simulink model "Grid_SensorLayout_SpatialAllignment_Clustering"  (R2018a)
settings: Solver=FixedStepAuto  StartTime=0.0  StopTime=SimulationTime  FixedStep=SamplingTime  RelTol=1e-3
values from neighbouring files (symbols this model uses):
  ValidateGRID = true    [SensorFusion_Script0_main.m]
  ValidateLAYOUT = true    [SensorFusion_Script0_main.m]
  VisualizeCLUSTERING = true    [SensorFusion_Script0_main.m]
undefined symbols (not defined in the file or in its folder): ACTIVATE_CAM, ACTIVATE_RAD, CAM1_detTimeStamp, CAM1_MeasNoise, CAM1_objClassID, CAM1_PX, CAM1_PY, CAM1_VX, CAM1_VY, CAM2_detTimeStamp, CAM2_MeasNoise, CAM2_objClassID, CAM2_PX, CAM2_PY, CAM2_VX, CAM2_VY, CAM3_detTimeStamp, CAM3_MeasNoise, CAM3_objClassID, CAM3_PX, CAM3_PY, CAM3_VX, CAM3_VY, CAM4_detTimeStamp, CAM4_MeasNoise, CAM4_objClassID, CAM4_PX, CAM4_PY, CAM4_VX, CAM4_VY, CAM5_detTimeStamp, CAM5_MeasNoise, CAM5_objClassID, CAM5_PX, CAM5_PY, CAM5_VX, CAM5_VY, CAM6_detTimeStamp, CAM6_MeasNoise, CAM6_objClassID, CAM6_PX, CAM6_PY, CAM6_VX, CAM6_VY, CAM7_detTimeStamp, CAM7_MeasNoise, CAM7_objClassID, CAM7_PX, CAM7_PY, CAM7_VX, CAM7_VY, CAM8_detTimeStamp, CAM8_MeasNoise, CAM8_objClassID, CAM8_PX, CAM8_PY, CAM8_VX, CAM8_VY, CAM_nMeas, CAM_TYPE ... (+171)
libraries: simulink_extras x4
(part 6 of 10)

== system Grid_SensorLayout_SpatialAllignment_Clustering/SENSOR_MEASUREMENTS/RADAR_CAMERA_EGO_SENSOR_INTERFACE/RadarSensors/Radar4/Subsystem ==
  SensorData : Inport
  px : Inport  Port=2
  py : Inport  Port=3
  vx : Inport  Port=4
  vy : Inport  Port=5
  id : Inport  Port=6
  SNR : Inport  Port=7
  NOISE_COV : Inport  Port=8
  TIME_STAMP : Inport  Port=9
  iter : Inport  Port=10
  Assignment : Assignment  DiagnosticForDimensions=Warning  IndexOptions=Index vector (port)  Indices=1  OutputSizes=1
  Bus Creator1 : BusCreator  Inputs=12  OutDataTypeStr=Bus: RadarMeasParam  NonVirtualBus=on
  Bus Creator2 : BusCreator  Inputs=12  OutDataTypeStr=Bus: RadarMeasParam  NonVirtualBus=on
  Constant{,1..5,8} (7 alike) : Constant  Value=single(0)
  Constant10 : Constant  Value=single(zeros(4,4))
  Constant13 : Constant  Value=single(10)
  Constant14 : Constant  Value=uint8(4)
  Constant16 : Constant  Value=int16(-1)
  Constant17 : Constant  Value=boolean(0)  OutDataTypeStr=boolean
  Constant6 : Constant  Value=uint8(4)
  Constant7 : Constant  Value=int16(0)
  Constant9 : Constant  Value=boolean(0)  OutDataTypeStr=boolean
  Switch : Switch  Criteria=u2 ~= 0
  R4 : Outport
  wires:
  Switch/1 -> Assignment/2
  Bus Creator2/1 -> Switch/1
  Bus Creator1/1 -> Switch/3
  Assignment/1 -> R4/1
  Constant5/1 -> Bus Creator1/9  "SNR"
  iter/1 -> Assignment/3
  id/1 -> Bus Creator1/2, Bus Creator2/2, Switch/2  "measID"
  SensorData/1 -> Assignment/1
  Constant3/1 -> Bus Creator1/7  "vy"
  Constant2/1 -> Bus Creator1/6  "vx"
  Constant1/1 -> Bus Creator1/5  "py"
  Constant/1 -> Bus Creator1/4  "px"
  Constant6/1 -> Bus Creator1/3  "radarID"
  TIME_STAMP/1 -> Bus Creator2/1  "TimeStamp"
  Constant14/1 -> Bus Creator2/3  "radarID"
  px/1 -> Bus Creator2/4  "px"
  py/1 -> Bus Creator2/5  "py"
  vx/1 -> Bus Creator2/6  "vx"
  vy/1 -> Bus Creator2/7  "vy"
  NOISE_COV/1 -> Bus Creator2/8  "NoiseCovarience"
  SNR/1 -> Bus Creator2/9  "SNR"
  Constant17/1 -> Bus Creator2/12  "StationaryFlag"
  Constant13/1 -> Bus Creator2/11  "measConfidence"
  Constant16/1 -> Bus Creator2/10  "Classification"
  Constant9/1 -> Bus Creator1/12  "StationaryFlag"
  Constant4/1 -> Bus Creator1/11  "measConfidence"
  Constant7/1 -> Bus Creator1/10  "Classification"
  Constant8/1 -> Bus Creator1/1  "TimeStamp"
  Constant10/1 -> Bus Creator1/8  "NoiseCovarience"

== system Grid_SensorLayout_SpatialAllignment_Clustering/SENSOR_MEASUREMENTS/RADAR_CAMERA_EGO_SENSOR_INTERFACE/RadarSensors/Radar5/ExtractMeasParam ==
  idx : Inport
  time : Inport  Port=2
  Constant : Constant  Value=RAD5_PX
  Constant1 : Constant  Value=RAD5_PY
  Constant2 : Constant  Value=RAD5_VX
  Constant3 : Constant  Value=RAD5_VY
  Constant4 : Constant  Value=RAD5_SNR
  Constant5 : Constant  Value=RAD5_MeasNoise
  Constant6 : Constant  Value=RAD5_detTimeStamp
  MeasNoise : Selector  NumberOfDimensions=4  InputPortWidth=3  IndexOptions=Index vector (port),Select all,Select all,Index vector (port)  Indices=[1 3],1,1,1  OutputSizes=1,1,1,1
  PosX : Selector  NumberOfDimensions=2  InputPortWidth=3  IndexOptions=Index vector (port),Index vector (port)  Indices=[1 3],1  OutputSizes=1,1
  PosY : Selector  NumberOfDimensions=2  InputPortWidth=3  IndexOptions=Index vector (port),Index vector (port)  Indices=[1 3],1  OutputSizes=1,1
  Reshape : Reshape  OutputDimensionality=Customize  OutputDimensions=[4,4]
  VelX : Selector  NumberOfDimensions=2  InputPortWidth=3  IndexOptions=Index vector (port),Index vector (port)  Indices=[1 3],1  OutputSizes=1,1
  VelY : Selector  NumberOfDimensions=2  InputPortWidth=3  IndexOptions=Index vector (port),Index vector (port)  Indices=[1 3],1  OutputSizes=1,1
  snr : Selector  NumberOfDimensions=2  InputPortWidth=3  IndexOptions=Index vector (port),Index vector (port)  Indices=[1 3],1  OutputSizes=1,1
  timeStamp : Selector  NumberOfDimensions=2  InputPortWidth=3  IndexOptions=Select all,Index vector (port)  Indices=[1 3],1  OutputSizes=1,1
  PX : Outport
  PY : Outport  Port=2
  VX : Outport  Port=3
  VY : Outport  Port=4
  SNR : Outport  Port=5
  NOISE_COV : Outport  Port=6
  measCaptureTime : Outport  Port=7
  wires:
  Constant3/1 -> VelY/1
  Constant2/1 -> VelX/1
  VelY/1 -> VY/1
  Constant/1 -> PosX/1
  idx/1 -> MeasNoise/3, snr/3, VelY/3, VelX/3, PosY/3, PosX/3
  Constant1/1 -> PosY/1
  VelX/1 -> VX/1
  PosX/1 -> PX/1
  PosY/1 -> PY/1
  time/1 -> timeStamp/2, MeasNoise/2, snr/2, VelY/2, VelX/2, PosY/2, PosX/2
  Constant4/1 -> snr/1
  snr/1 -> SNR/1
  Constant5/1 -> MeasNoise/1
  Constant6/1 -> timeStamp/1
  MeasNoise/1 -> Reshape/1
  timeStamp/1 -> measCaptureTime/1
  Reshape/1 -> NOISE_COV/1

== system Grid_SensorLayout_SpatialAllignment_Clustering/SENSOR_MEASUREMENTS/RADAR_CAMERA_EGO_SENSOR_INTERFACE/RadarSensors/Radar5/IsValid1 ==
  idx : Inport
  px : Inport  Port=2
  py : Inport  Port=3
  vx : Inport  Port=4
  vy : Inport  Port=5
  Abs{,1..3} (4 alike) : Abs
  Add : Sum  Inputs=++++
  Constant : Constant  Value=uint16(0)
  Data Type Conversion : DataTypeConversion  OutDataTypeStr=uint16
  Switch : Switch  Threshold=0.0001
  ID : Outport
  wires:
  Add/1 -> Switch/2
  Abs2/1 -> Add/3
  Constant/1 -> Switch/3
  Abs/1 -> Add/1
  px/1 -> Abs/1
  Abs3/1 -> Add/4
  Abs1/1 -> Add/2
  vy/1 -> Abs3/1
  py/1 -> Abs1/1
  vx/1 -> Abs2/1
  idx/1 -> Data Type Conversion/1
  Switch/1 -> ID/1
  Data Type Conversion/1 -> Switch/1

== system Grid_SensorLayout_SpatialAllignment_Clustering/SENSOR_MEASUREMENTS/RADAR_CAMERA_EGO_SENSOR_INTERFACE/RadarSensors/Radar5/Subsystem ==
  SensorData : Inport
  px : Inport  Port=2
  py : Inport  Port=3
  vx : Inport  Port=4
  vy : Inport  Port=5
  id : Inport  Port=6
  SNR : Inport  Port=7
  NOISE_COV : Inport  Port=8
  TIME_STAMP : Inport  Port=9
  iter : Inport  Port=10
  Assignment : Assignment  DiagnosticForDimensions=Warning  IndexOptions=Index vector (port)  Indices=1  OutputSizes=1
  Bus Creator1 : BusCreator  Inputs=12  OutDataTypeStr=Bus: RadarMeasParam  NonVirtualBus=on
  Bus Creator2 : BusCreator  Inputs=12  OutDataTypeStr=Bus: RadarMeasParam  NonVirtualBus=on
  Constant{,1..5,8} (7 alike) : Constant  Value=single(0)
  Constant10 : Constant  Value=single(zeros(4,4))
  Constant13 : Constant  Value=single(10)
  Constant14 : Constant  Value=uint8(5)
  Constant16 : Constant  Value=int16(-1)
  Constant17 : Constant  Value=boolean(0)  OutDataTypeStr=boolean
  Constant6 : Constant  Value=uint8(5)
  Constant7 : Constant  Value=int16(0)
  Constant9 : Constant  Value=boolean(0)  OutDataTypeStr=boolean
  Switch : Switch  Criteria=u2 ~= 0
  R5 : Outport
  wires:
  Switch/1 -> Assignment/2
  Bus Creator2/1 -> Switch/1
  Bus Creator1/1 -> Switch/3
  Assignment/1 -> R5/1
  Constant5/1 -> Bus Creator1/9  "SNR"
  iter/1 -> Assignment/3
  id/1 -> Bus Creator1/2, Bus Creator2/2, Switch/2  "measID"
  SensorData/1 -> Assignment/1
  Constant3/1 -> Bus Creator1/7  "vy"
  Constant2/1 -> Bus Creator1/6  "vx"
  Constant1/1 -> Bus Creator1/5  "py"
  Constant/1 -> Bus Creator1/4  "px"
  Constant6/1 -> Bus Creator1/3  "radarID"
  TIME_STAMP/1 -> Bus Creator2/1  "TimeStamp"
  Constant14/1 -> Bus Creator2/3  "radarID"
  px/1 -> Bus Creator2/4  "px"
  py/1 -> Bus Creator2/5  "py"
  vx/1 -> Bus Creator2/6  "vx"
  vy/1 -> Bus Creator2/7  "vy"
  NOISE_COV/1 -> Bus Creator2/8  "NoiseCovarience"
  SNR/1 -> Bus Creator2/9  "SNR"
  Constant17/1 -> Bus Creator2/12  "StationaryFlag"
  Constant13/1 -> Bus Creator2/11  "measConfidence"
  Constant16/1 -> Bus Creator2/10  "Classification"
  Constant9/1 -> Bus Creator1/12  "StationaryFlag"
  Constant4/1 -> Bus Creator1/11  "measConfidence"
  Constant7/1 -> Bus Creator1/10  "Classification"
  Constant8/1 -> Bus Creator1/1  "TimeStamp"
  Constant10/1 -> Bus Creator1/8  "NoiseCovarience"

== system Grid_SensorLayout_SpatialAllignment_Clustering/SENSOR_MEASUREMENTS/RADAR_CAMERA_EGO_SENSOR_INTERFACE/RadarSensors/Radar6/ExtractMeasParam ==
  idx : Inport
  time : Inport  Port=2
  Constant : Constant  Value=RAD6_PX
  Constant1 : Constant  Value=RAD6_PY
  Constant2 : Constant  Value=RAD6_VX
  Constant3 : Constant  Value=RAD6_VY
  Constant4 : Constant  Value=RAD6_SNR
  Constant5 : Constant  Value=RAD6_MeasNoise
  Constant6 : Constant  Value=RAD6_detTimeStamp
  MeasNoise : Selector  NumberOfDimensions=4  InputPortWidth=3  IndexOptions=Index vector (port),Select all,Select all,Index vector (port)  Indices=[1 3],1,1,1  OutputSizes=1,1,1,1
  PosX : Selector  NumberOfDimensions=2  InputPortWidth=3  IndexOptions=Index vector (port),Index vector (port)  Indices=[1 3],1  OutputSizes=1,1
  PosY : Selector  NumberOfDimensions=2  InputPortWidth=3  IndexOptions=Index vector (port),Index vector (port)  Indices=[1 3],1  OutputSizes=1,1
  Reshape : Reshape  OutputDimensionality=Customize  OutputDimensions=[4,4]
  VelX : Selector  NumberOfDimensions=2  InputPortWidth=3  IndexOptions=Index vector (port),Index vector (port)  Indices=[1 3],1  OutputSizes=1,1
  VelY : Selector  NumberOfDimensions=2  InputPortWidth=3  IndexOptions=Index vector (port),Index vector (port)  Indices=[1 3],1  OutputSizes=1,1
  snr : Selector  NumberOfDimensions=2  InputPortWidth=3  IndexOptions=Index vector (port),Index vector (port)  Indices=[1 3],1  OutputSizes=1,1
  timeStamp : Selector  NumberOfDimensions=2  InputPortWidth=3  IndexOptions=Select all,Index vector (port)  Indices=[1 3],1  OutputSizes=1,1
  PX : Outport
  PY : Outport  Port=2
  VX : Outport  Port=3
  VY : Outport  Port=4
  SNR : Outport  Port=5
  NOISE_COV : Outport  Port=6
  measCaptureTime : Outport  Port=7
  wires:
  Constant3/1 -> VelY/1
  Constant2/1 -> VelX/1
  VelY/1 -> VY/1
  Constant/1 -> PosX/1
  idx/1 -> MeasNoise/3, snr/3, VelY/3, VelX/3, PosY/3, PosX/3
  Constant1/1 -> PosY/1
  VelX/1 -> VX/1
  PosX/1 -> PX/1
  PosY/1 -> PY/1
  time/1 -> timeStamp/2, MeasNoise/2, snr/2, VelY/2, VelX/2, PosY/2, PosX/2
  Constant4/1 -> snr/1
  snr/1 -> SNR/1
  Constant5/1 -> MeasNoise/1
  Constant6/1 -> timeStamp/1
  MeasNoise/1 -> Reshape/1
  timeStamp/1 -> measCaptureTime/1
  Reshape/1 -> NOISE_COV/1

== system Grid_SensorLayout_SpatialAllignment_Clustering/SENSOR_MEASUREMENTS/RADAR_CAMERA_EGO_SENSOR_INTERFACE/RadarSensors/Radar6/IsValid1 ==
  idx : Inport
  px : Inport  Port=2
  py : Inport  Port=3
  vx : Inport  Port=4
  vy : Inport  Port=5
  Abs{,1..3} (4 alike) : Abs
  Add : Sum  Inputs=++++
  Constant : Constant  Value=uint16(0)
  Data Type Conversion : DataTypeConversion  OutDataTypeStr=uint16
  Switch : Switch  Threshold=0.0001
  ID : Outport
  wires:
  Add/1 -> Switch/2
  Abs2/1 -> Add/3
  Constant/1 -> Switch/3
  Abs/1 -> Add/1
  px/1 -> Abs/1
  Abs3/1 -> Add/4
  Abs1/1 -> Add/2
  vy/1 -> Abs3/1
  py/1 -> Abs1/1
  vx/1 -> Abs2/1
  idx/1 -> Data Type Conversion/1
  Switch/1 -> ID/1
  Data Type Conversion/1 -> Switch/1

== system Grid_SensorLayout_SpatialAllignment_Clustering/SENSOR_MEASUREMENTS/RADAR_CAMERA_EGO_SENSOR_INTERFACE/RadarSensors/Radar6/Subsystem ==
  SensorData : Inport
  px : Inport  Port=2
  py : Inport  Port=3
  vx : Inport  Port=4
  vy : Inport  Port=5
  id : Inport  Port=6
  SNR : Inport  Port=7
  NOISE_COV : Inport  Port=8
  TIME_STAMP : Inport  Port=9
  iter : Inport  Port=10
  Assignment : Assignment  DiagnosticForDimensions=Warning  IndexOptions=Index vector (port)  Indices=1  OutputSizes=1
  Bus Creator1 : BusCreator  Inputs=12  OutDataTypeStr=Bus: RadarMeasParam  NonVirtualBus=on
  Bus Creator2 : BusCreator  Inputs=12  OutDataTypeStr=Bus: RadarMeasParam  NonVirtualBus=on
  Constant{,1..5,8} (7 alike) : Constant  Value=single(0)
  Constant10 : Constant  Value=single(zeros(4,4))
  Constant13 : Constant  Value=single(10)
  Constant14 : Constant  Value=uint8(6)
  Constant16 : Constant  Value=int16(-1)
  Constant17 : Constant  Value=boolean(0)  OutDataTypeStr=boolean
  Constant6 : Constant  Value=uint8(6)
  Constant7 : Constant  Value=int16(0)
  Constant9 : Constant  Value=boolean(0)  OutDataTypeStr=boolean
  Switch : Switch  Criteria=u2 ~= 0
  R6 : Outport
  wires:
  Switch/1 -> Assignment/2
  Bus Creator2/1 -> Switch/1
  Bus Creator1/1 -> Switch/3
  Assignment/1 -> R6/1
  Constant5/1 -> Bus Creator1/9  "SNR"
  iter/1 -> Assignment/3
  id/1 -> Bus Creator1/2, Bus Creator2/2, Switch/2  "measID"
  SensorData/1 -> Assignment/1
  Constant3/1 -> Bus Creator1/7  "vy"
  Constant2/1 -> Bus Creator1/6  "vx"
  Constant1/1 -> Bus Creator1/5  "py"
  Constant/1 -> Bus Creator1/4  "px"
  Constant6/1 -> Bus Creator1/3  "radarID"
  TIME_STAMP/1 -> Bus Creator2/1  "TimeStamp"
  Constant14/1 -> Bus Creator2/3  "radarID"
  px/1 -> Bus Creator2/4  "px"
  py/1 -> Bus Creator2/5  "py"
  vx/1 -> Bus Creator2/6  "vx"
  vy/1 -> Bus Creator2/7  "vy"
  NOISE_COV/1 -> Bus Creator2/8  "NoiseCovarience"
  SNR/1 -> Bus Creator2/9  "SNR"
  Constant17/1 -> Bus Creator2/12  "StationaryFlag"
  Constant13/1 -> Bus Creator2/11  "measConfidence"
  Constant16/1 -> Bus Creator2/10  "Classification"
  Constant9/1 -> Bus Creator1/12  "StationaryFlag"
  Constant4/1 -> Bus Creator1/11  "measConfidence"
  Constant7/1 -> Bus Creator1/10  "Classification"
  Constant8/1 -> Bus Creator1/1  "TimeStamp"
  Constant10/1 -> Bus Creator1/8  "NoiseCovarience"

== system Grid_SensorLayout_SpatialAllignment_Clustering/SENSOR_MEASUREMENTS/RADAR_CAMERA_EGO_SENSOR_INTERFACE/RoadSensors/LineSensor1/CHECK_IF_DATA_IS_VALID ==
  LineID : Inport
  curvature : Inport  Port=2
  curvatureRate : Inport  Port=3
  curvLength : Inport  Port=4
  HeadingAngle : Inport  Port=5
  Abs{,1..3} (4 alike) : Abs
  Add : Sum  Inputs=++++
  Constant : Constant  Value=uint16(0)
  Data Type Conversion : DataTypeConversion  OutDataTypeStr=uint16
  Switch : Switch  Threshold=0.000001
  validID : Outport
  wires:
  Add/1 -> Switch/2
  Abs2/1 -> Add/3
  Constant/1 -> Switch/3
  Abs/1 -> Add/1
  curvature/1 -> Abs/1
  Abs3/1 -> Add/4
  Abs1/1 -> Add/2
  HeadingAngle/1 -> Abs3/1
  curvatureRate/1 -> Abs1/1
  curvLength/1 -> Abs2/1
  LineID/1 -> Data Type Conversion/1
  Switch/1 -> validID/1
  Data Type Conversion/1 -> Switch/1

== system Grid_SensorLayout_SpatialAllignment_Clustering/SENSOR_MEASUREMENTS/RADAR_CAMERA_EGO_SENSOR_INTERFACE/RoadSensors/LineSensor1/GET_DATA ==
  idx : Inport
  time : Inport  Port=2
  Constant : Constant  Value=LINE_CURVATURE_CAM1
  Constant1 : Constant  Value=LINE_CURVDERIVATIVE_CAM1
  Constant2 : Constant  Value=LINE_CURVELENGTH_CAM1
  Constant3 : Constant  Value=LINE_HEADINGANGLE_CAM1
  Constant4 : Constant  Value=LINE_LATERALOFFSET_CAM1
  Constant5 : Constant  Value=LINE_XMIN_CAM1
  Constant6 : Constant  Value=LINE_detTimeStamp_CAM1
  Constant7 : Constant  Value=LINE_XMAX_CAM1
  Constant8 : Constant  Value=LINE_WIDTH_CAM1
  CurvLength : Selector  NumberOfDimensions=2  InputPortWidth=3  IndexOptions=Index vector (port),Index vector (port)  Indices=[1 3],1  OutputSizes=1,1
  Curvature : Selector  NumberOfDimensions=2  InputPortWidth=3  IndexOptions=Index vector (port),Index vector (port)  Indices=[1 3],1  OutputSizes=1,1
  CurvatureRate : Selector  NumberOfDimensions=2  InputPortWidth=3  IndexOptions=Index vector (port),Index vector (port)  Indices=[1 3],1  OutputSizes=1,1
  HeadingAngle : Selector  NumberOfDimensions=2  InputPortWidth=3  IndexOptions=Index vector (port),Index vector (port)  Indices=[1 3],1  OutputSizes=1,1
  LateralOffset : Selector  NumberOfDimensions=2  InputPortWidth=3  IndexOptions=Index vector (port),Index vector (port)  Indices=[1 3],1  OutputSizes=1,1
  lineWidth : Selector  NumberOfDimensions=2  InputPortWidth=3  IndexOptions=Index vector (port),Index vector (port)  Indices=[1 3],1  OutputSizes=1,1
  minValidX : Selector  NumberOfDimensions=2  InputPortWidth=3  IndexOptions=Index vector (port),Index vector (port)  Indices=[1 3],1  OutputSizes=1,1
  minValidY : Selector  NumberOfDimensions=2  InputPortWidth=3  IndexOptions=Index vector (port),Index vector (port)  Indices=[1 3],1  OutputSizes=1,1
  timeStamp : Selector  NumberOfDimensions=2  InputPortWidth=3  IndexOptions=Select all,Index vector (port)  Indices=[1 3],1  OutputSizes=1,1
  curvature : Outport
  curvRate : Outport  Port=2
  curvLength : Outport  Port=3
  headingAngle : Outport  Port=4
  lateralOffset : Outport  Port=5
  xmin : Outport  Port=6
  xmax : Outport  Port=7
  lineMarkWidth : Outport  Port=8
  measCaptureTime : Outport  Port=9
  wires:
  Constant3/1 -> HeadingAngle/1
  Constant2/1 -> CurvLength/1
  HeadingAngle/1 -> headingAngle/1
  Constant/1 -> Curvature/1
  Constant1/1 -> CurvatureRate/1
  CurvLength/1 -> curvLength/1
  Curvature/1 -> curvature/1
  CurvatureRate/1 -> curvRate/1
  Constant4/1 -> LateralOffset/1
  Constant5/1 -> minValidX/1
  Constant6/1 -> timeStamp/1
  timeStamp/1 -> measCaptureTime/1
  minValidX/1 -> xmin/1
  LateralOffset/1 -> lateralOffset/1
  minValidY/1 -> xmax/1
  Constant7/1 -> minValidY/1
  lineWidth/1 -> lineMarkWidth/1
  time/1 -> minValidX/2, minValidY/2, lineWidth/2, timeStamp/2, LateralOffset/2, HeadingAngle/2, CurvLength/2, CurvatureRate/2, Curvature/2
  idx/1 -> minValidX/3, lineWidth/3, minValidY/3, LateralOffset/3, HeadingAngle/3, CurvLength/3, CurvatureRate/3, Curvature/3
  Constant8/1 -> lineWidth/1

== system Grid_SensorLayout_SpatialAllignment_Clustering/SENSOR_MEASUREMENTS/RADAR_CAMERA_EGO_SENSOR_INTERFACE/RoadSensors/LineSensor1/SET_DATA ==
  CameraLineCoeff : Inport
  curv : Inport  Port=2
  curvRate : Inport  Port=3
  curvLen : Inport  Port=4
  alpha : Inport  Port=5
  ValidID : Inport  Port=6
  lateralOffset : Inport  Port=7
  xmin : Inport  Port=8
  xmax : Inport  Port=9
  lineWidth : Inport  Port=10
  TIME_STAMP : Inport  Port=11
  iter : Inport  Port=12
  Assignment : Assignment  DiagnosticForDimensions=Warning  IndexOptions=Index vector (port)  Indices=1  OutputSizes=1
  Bus Creator1 : BusCreator  Inputs=11  OutDataTypeStr=Bus: LineMeasParam  NonVirtualBus=on
  Bus Creator2 : BusCreator  Inputs=11  OutDataTypeStr=Bus: LineMeasParam  NonVirtualBus=on
  Constant1 : Constant  Value=single(10)
  Constant14 : Constant  Value=uint8(1)
  Constant2 : Constant  Value=single(10)
  Constant{35..39,43} (6 alike) : Constant  Value=single(0)
  Constant44 : Constant  Value=single(10)
  Switch : Switch  Criteria=u2 ~= 0
  C1 : Outport
  wires:
  Bus Creator1/1 -> Switch/3
  ValidID/1 -> Bus Creator1/2, Switch/2, Bus Creator2/2  "lineID"
  Bus Creator2/1 -> Switch/1
  CameraLineCoeff/1 -> Assignment/1
  Switch/1 -> Assignment/2
  iter/1 -> Assignment/3
  Assignment/1 -> C1/1
  TIME_STAMP/1 -> Bus Creator2/1  "TimeStamp"
  curv/1 -> Bus Creator2/4  "curvature"
  curvRate/1 -> Bus Creator2/5  "curvatureRate"
  curvLen/1 -> Bus Creator2/6  "curveLength"
  alpha/1 -> Bus Creator2/7  "HeadingAngle"
  lateralOffset/1 -> Bus Creator2/8  "LateralOffset"
  lineWidth/1 -> Bus Creator2/11  "LineMarkWidth"
  xmax/1 -> Bus Creator2/10  "validMinLongCoordLine"
  xmin/1 -> Bus Creator2/9  "validMaxLongCoordLine"
  Constant35/1 -> Bus Creator1/1  "TimeStamp"
  Constant14/1 -> Bus Creator2/3, Bus Creator1/3  "cameraID"
  Constant36/1 -> Bus Creator1/4  "curvature"
  Constant37/1 -> Bus Creator1/5  "curvatureRate"
  Constant38/1 -> Bus Creator1/6  "curveLength"
  Constant39/1 -> Bus Creator1/7  "HeadingAngle"
  Constant43/1 -> Bus Creator1/8  "LateralOffset"
  Constant44/1 -> Bus Creator1/9  "validMaxLongCoordLine"
  Constant1/1 -> Bus Creator1/10  "validMinLongCoordLine"
  Constant2/1 -> Bus Creator1/11  "LineMarkWidth"

== system Grid_SensorLayout_SpatialAllignment_Clustering/SENSOR_MEASUREMENTS/RADAR_CAMERA_EGO_SENSOR_INTERFACE/RoadSensors/LineSensor2/ExtractMeasParam1 ==
  idx : Inport
  time : Inport  Port=2
  Constant : Constant  Value=LINE_CURVATURE_CAM2
  Constant1 : Constant  Value=LINE_CURVDERIVATIVE_CAM2
  Constant2 : Constant  Value=LINE_CURVELENGTH_CAM2
  Constant3 : Constant  Value=LINE_HEADINGANGLE_CAM2
  Constant4 : Constant  Value=LINE_LATERALOFFSET_CAM2
  Constant5 : Constant  Value=LINE_XMIN_CAM2
  Constant6 : Constant  Value=LINE_detTimeStamp_CAM2
  Constant7 : Constant  Value=LINE_XMAX_CAM2
  Constant8 : Constant  Value=LINE_WIDTH_CAM2
  CurvLength : Selector  NumberOfDimensions=2  InputPortWidth=3  IndexOptions=Index vector (port),Index vector (port)  Indices=[1 3],1  OutputSizes=1,1
  Curvature : Selector  NumberOfDimensions=2  InputPortWidth=3  IndexOptions=Index vector (port),Index vector (port)  Indices=[1 3],1  OutputSizes=1,1
  CurvatureRate : Selector  NumberOfDimensions=2  InputPortWidth=3  IndexOptions=Index vector (port),Index vector (port)  Indices=[1 3],1  OutputSizes=1,1
  HeadingAngle : Selector  NumberOfDimensions=2  InputPortWidth=3  IndexOptions=Index vector (port),Index vector (port)  Indices=[1 3],1  OutputSizes=1,1
  LateralOffset : Selector  NumberOfDimensions=2  InputPortWidth=3  IndexOptions=Index vector (port),Index vector (port)  Indices=[1 3],1  OutputSizes=1,1
  lineWidth : Selector  NumberOfDimensions=2  InputPortWidth=3  IndexOptions=Index vector (port),Index vector (port)  Indices=[1 3],1  OutputSizes=1,1
  minValidX : Selector  NumberOfDimensions=2  InputPortWidth=3  IndexOptions=Index vector (port),Index vector (port)  Indices=[1 3],1  OutputSizes=1,1
  minValidY : Selector  NumberOfDimensions=2  InputPortWidth=3  IndexOptions=Index vector (port),Index vector (port)  Indices=[1 3],1  OutputSizes=1,1
  timeStamp : Selector  NumberOfDimensions=2  InputPortWidth=3  IndexOptions=Select all,Index vector (port)  Indices=[1 3],1  OutputSizes=1,1
  curvature : Outport
  curvRate : Outport  Port=2
  curvLength : Outport  Port=3
  headingAngle : Outport  Port=4
  lateralOffset : Outport  Port=5
  xmin : Outport  Port=6
  xmax : Outport  Port=7
  lineMarkWidth : Outport  Port=8
  measCaptureTime : Outport  Port=9
  wires:
  Constant3/1 -> HeadingAngle/1
  Constant2/1 -> CurvLength/1
  HeadingAngle/1 -> headingAngle/1
  Constant/1 -> Curvature/1
  Constant1/1 -> CurvatureRate/1
  CurvLength/1 -> curvLength/1
  Curvature/1 -> curvature/1
  CurvatureRate/1 -> curvRate/1
  Constant4/1 -> LateralOffset/1
  Constant5/1 -> minValidX/1
  Constant6/1 -> timeStamp/1
  timeStamp/1 -> measCaptureTime/1
  minValidX/1 -> xmin/1
  LateralOffset/1 -> lateralOffset/1
  minValidY/1 -> xmax/1
  Constant7/1 -> minValidY/1
  lineWidth/1 -> lineMarkWidth/1
  time/1 -> minValidX/2, minValidY/2, lineWidth/2, timeStamp/2, LateralOffset/2, HeadingAngle/2, CurvLength/2, CurvatureRate/2, Curvature/2
  idx/1 -> minValidX/3, lineWidth/3, minValidY/3, LateralOffset/3, HeadingAngle/3, CurvLength/3, CurvatureRate/3, Curvature/3
  Constant8/1 -> lineWidth/1

== system Grid_SensorLayout_SpatialAllignment_Clustering/SENSOR_MEASUREMENTS/RADAR_CAMERA_EGO_SENSOR_INTERFACE/RoadSensors/LineSensor2/IsValid2 ==
  LineID : Inport
  curvature : Inport  Port=2
  curvatureRate : Inport  Port=3
  curvLength : Inport  Port=4
  HeadingAngle : Inport  Port=5
  Abs{,1..3} (4 alike) : Abs
  Add : Sum  Inputs=++++
  Constant : Constant  Value=uint16(0)
  Data Type Conversion : DataTypeConversion  OutDataTypeStr=uint16
  Switch : Switch  Threshold=0.000001
  validID : Outport
  wires:
  Add/1 -> Switch/2
  Abs2/1 -> Add/3
  Constant/1 -> Switch/3
  Abs/1 -> Add/1
  curvature/1 -> Abs/1
  Abs3/1 -> Add/4
  Abs1/1 -> Add/2
  HeadingAngle/1 -> Abs3/1
  curvatureRate/1 -> Abs1/1
  curvLength/1 -> Abs2/1
  LineID/1 -> Data Type Conversion/1
  Switch/1 -> validID/1
  Data Type Conversion/1 -> Switch/1

== system Grid_SensorLayout_SpatialAllignment_Clustering/SENSOR_MEASUREMENTS/RADAR_CAMERA_EGO_SENSOR_INTERFACE/RoadSensors/LineSensor2/Subsystem1 ==
  CameraLineCoeff : Inport
  curv : Inport  Port=2
  curvRate : Inport  Port=3
  curvLen : Inport  Port=4
  alpha : Inport  Port=5
  ValidID : Inport  Port=6
  lateralOffset : Inport  Port=7
  xmin : Inport  Port=8
  xmax : Inport  Port=9
  lineWidth : Inport  Port=10
  TIME_STAMP : Inport  Port=11
  iter : Inport  Port=12
  Assignment : Assignment  DiagnosticForDimensions=Warning  IndexOptions=Index vector (port)  Indices=1  OutputSizes=1
  Bus Creator1 : BusCreator  Inputs=11  OutDataTypeStr=Bus: LineMeasParam  NonVirtualBus=on
  Bus Creator2 : BusCreator  Inputs=11  OutDataTypeStr=Bus: LineMeasParam  NonVirtualBus=on
  Constant1 : Constant  Value=single(10)
  Constant14 : Constant  Value=uint8(2)
  Constant2 : Constant  Value=single(10)
  Constant{35..39,43} (6 alike) : Constant  Value=single(0)
  Constant44 : Constant  Value=single(10)
  Switch : Switch  Criteria=u2 ~= 0
  C1 : Outport
  wires:
  Bus Creator1/1 -> Switch/3
  ValidID/1 -> Bus Creator1/2, Switch/2, Bus Creator2/2  "lineID"
  Bus Creator2/1 -> Switch/1
  CameraLineCoeff/1 -> Assignment/1
  Switch/1 -> Assignment/2
  iter/1 -> Assignment/3
  Assignment/1 -> C1/1
  TIME_STAMP/1 -> Bus Creator2/1  "TimeStamp"
  curv/1 -> Bus Creator2/4  "curvature"
  curvRate/1 -> Bus Creator2/5  "curvatureRate"
  curvLen/1 -> Bus Creator2/6  "curveLength"
  alpha/1 -> Bus Creator2/7  "HeadingAngle"
  lateralOffset/1 -> Bus Creator2/8  "LateralOffset"
  lineWidth/1 -> Bus Creator2/11  "LineMarkWidth"
  xmax/1 -> Bus Creator2/10  "validMinLongCoordLine"
  xmin/1 -> Bus Creator2/9  "validMaxLongCoordLine"
  Constant35/1 -> Bus Creator1/1  "TimeStamp"
  Constant14/1 -> Bus Creator2/3, Bus Creator1/3  "cameraID"
  Constant36/1 -> Bus Creator1/4  "curvature"
  Constant37/1 -> Bus Creator1/5  "curvatureRate"
  Constant38/1 -> Bus Creator1/6  "curveLength"
  Constant39/1 -> Bus Creator1/7  "HeadingAngle"
  Constant43/1 -> Bus Creator1/8  "LateralOffset"
  Constant44/1 -> Bus Creator1/9  "validMaxLongCoordLine"
  Constant1/1 -> Bus Creator1/10  "validMinLongCoordLine"
  Constant2/1 -> Bus Creator1/11  "LineMarkWidth"

== system Grid_SensorLayout_SpatialAllignment_Clustering/SENSOR_MEASUREMENTS/RADAR_CAMERA_EGO_SENSOR_INTERFACE/RoadSensors/LineSensor3/ExtractMeasParam1 ==
  idx : Inport
  time : Inport  Port=2
  Constant : Constant  Value=LINE_CURVATURE_CAM3
  Constant1 : Constant  Value=LINE_CURVDERIVATIVE_CAM3
  Constant2 : Constant  Value=LINE_CURVELENGTH_CAM3
  Constant3 : Constant  Value=LINE_HEADINGANGLE_CAM3
  Constant4 : Constant  Value=LINE_LATERALOFFSET_CAM3
  Constant5 : Constant  Value=LINE_XMIN_CAM3
  Constant6 : Constant  Value=LINE_detTimeStamp_CAM3
  Constant7 : Constant  Value=LINE_XMAX_CAM3
  Constant8 : Constant  Value=LINE_WIDTH_CAM3
  CurvLength : Selector  NumberOfDimensions=2  InputPortWidth=3  IndexOptions=Index vector (port),Index vector (port)  Indices=[1 3],1  OutputSizes=1,1
  Curvature : Selector  NumberOfDimensions=2  InputPortWidth=3  IndexOptions=Index vector (port),Index vector (port)  Indices=[1 3],1  OutputSizes=1,1
  CurvatureRate : Selector  NumberOfDimensions=2  InputPortWidth=3  IndexOptions=Index vector (port),Index vector (port)  Indices=[1 3],1  OutputSizes=1,1
  HeadingAngle : Selector  NumberOfDimensions=2  InputPortWidth=3  IndexOptions=Index vector (port),Index vector (port)  Indices=[1 3],1  OutputSizes=1,1
  LateralOffset : Selector  NumberOfDimensions=2  InputPortWidth=3  IndexOptions=Index vector (port),Index vector (port)  Indices=[1 3],1  OutputSizes=1,1
  lineWidth : Selector  NumberOfDimensions=2  InputPortWidth=3  IndexOptions=Index vector (port),Index vector (port)  Indices=[1 3],1  OutputSizes=1,1
  minValidX : Selector  NumberOfDimensions=2  InputPortWidth=3  IndexOptions=Index vector (port),Index vector (port)  Indices=[1 3],1  OutputSizes=1,1
  minValidY : Selector  NumberOfDimensions=2  InputPortWidth=3  IndexOptions=Index vector (port),Index vector (port)  Indices=[1 3],1  OutputSizes=1,1
  timeStamp : Selector  NumberOfDimensions=2  InputPortWidth=3  IndexOptions=Select all,Index vector (port)  Indices=[1 3],1  OutputSizes=1,1
  curvature : Outport
  curvRate : Outport  Port=2
  curvLength : Outport  Port=3
  headingAngle : Outport  Port=4
  lateralOffset : Outport  Port=5
  xmin : Outport  Port=6
  xmax : Outport  Port=7
  lineMarkWidth : Outport  Port=8
  measCaptureTime : Outport  Port=9
  wires:
  Constant3/1 -> HeadingAngle/1
  Constant2/1 -> CurvLength/1
  HeadingAngle/1 -> headingAngle/1
  Constant/1 -> Curvature/1
  Constant1/1 -> CurvatureRate/1
  CurvLength/1 -> curvLength/1
  Curvature/1 -> curvature/1
  CurvatureRate/1 -> curvRate/1
  Constant4/1 -> LateralOffset/1
  Constant5/1 -> minValidX/1
  Constant6/1 -> timeStamp/1
  timeStamp/1 -> measCaptureTime/1
  minValidX/1 -> xmin/1
  LateralOffset/1 -> lateralOffset/1
  minValidY/1 -> xmax/1
  Constant7/1 -> minValidY/1
  lineWidth/1 -> lineMarkWidth/1
  time/1 -> minValidX/2, minValidY/2, lineWidth/2, timeStamp/2, LateralOffset/2, HeadingAngle/2, CurvLength/2, CurvatureRate/2, Curvature/2
  idx/1 -> minValidX/3, lineWidth/3, minValidY/3, LateralOffset/3, HeadingAngle/3, CurvLength/3, CurvatureRate/3, Curvature/3
  Constant8/1 -> lineWidth/1

== system Grid_SensorLayout_SpatialAllignment_Clustering/SENSOR_MEASUREMENTS/RADAR_CAMERA_EGO_SENSOR_INTERFACE/RoadSensors/LineSensor3/IsValid2 ==
  LineID : Inport
  curvature : Inport  Port=2
  curvatureRate : Inport  Port=3
  curvLength : Inport  Port=4
  HeadingAngle : Inport  Port=5
  Abs{,1..3} (4 alike) : Abs
  Add : Sum  Inputs=++++
  Constant : Constant  Value=uint16(0)
  Data Type Conversion : DataTypeConversion  OutDataTypeStr=uint16
  Switch : Switch  Threshold=0.000001
  validID : Outport
  wires:
  Add/1 -> Switch/2
  Abs2/1 -> Add/3
  Constant/1 -> Switch/3
  Abs/1 -> Add/1
  curvature/1 -> Abs/1
  Abs3/1 -> Add/4
  Abs1/1 -> Add/2
  HeadingAngle/1 -> Abs3/1
  curvatureRate/1 -> Abs1/1
  curvLength/1 -> Abs2/1
  LineID/1 -> Data Type Conversion/1
  Switch/1 -> validID/1
  Data Type Conversion/1 -> Switch/1

== system Grid_SensorLayout_SpatialAllignment_Clustering/SENSOR_MEASUREMENTS/RADAR_CAMERA_EGO_SENSOR_INTERFACE/RoadSensors/LineSensor3/Subsystem1 ==
  CameraLineCoeff : Inport
  curv : Inport  Port=2
  curvRate : Inport  Port=3
  curvLen : Inport  Port=4
  alpha : Inport  Port=5
  ValidID : Inport  Port=6
  lateralOffset : Inport  Port=7
  xmin : Inport  Port=8
  xmax : Inport  Port=9
  lineWidth : Inport  Port=10
  TIME_STAMP : Inport  Port=11
  iter : Inport  Port=12
  Assignment : Assignment  DiagnosticForDimensions=Warning  IndexOptions=Index vector (port)  Indices=1  OutputSizes=1
  Bus Creator1 : BusCreator  Inputs=11  OutDataTypeStr=Bus: LineMeasParam  NonVirtualBus=on
  Bus Creator2 : BusCreator  Inputs=11  OutDataTypeStr=Bus: LineMeasParam  NonVirtualBus=on
  Constant1 : Constant  Value=single(10)
  Constant14 : Constant  Value=uint8(3)
  Constant2 : Constant  Value=single(10)
  Constant{35..39,43} (6 alike) : Constant  Value=single(0)
  Constant44 : Constant  Value=single(10)
  Switch : Switch  Criteria=u2 ~= 0
  C1 : Outport
  wires:
  Bus Creator1/1 -> Switch/3
  ValidID/1 -> Bus Creator1/2, Switch/2, Bus Creator2/2  "lineID"
  Bus Creator2/1 -> Switch/1
  CameraLineCoeff/1 -> Assignment/1
  Switch/1 -> Assignment/2
  iter/1 -> Assignment/3
  Assignment/1 -> C1/1
  TIME_STAMP/1 -> Bus Creator2/1  "TimeStamp"
  curv/1 -> Bus Creator2/4  "curvature"
  curvRate/1 -> Bus Creator2/5  "curvatureRate"
  curvLen/1 -> Bus Creator2/6  "curveLength"
  alpha/1 -> Bus Creator2/7  "HeadingAngle"
  lateralOffset/1 -> Bus Creator2/8  "LateralOffset"
  lineWidth/1 -> Bus Creator2/11  "LineMarkWidth"
  xmax/1 -> Bus Creator2/10  "validMinLongCoordLine"
  xmin/1 -> Bus Creator2/9  "validMaxLongCoordLine"
  Constant35/1 -> Bus Creator1/1  "TimeStamp"
  Constant14/1 -> Bus Creator2/3, Bus Creator1/3  "cameraID"
  Constant36/1 -> Bus Creator1/4  "curvature"
  Constant37/1 -> Bus Creator1/5  "curvatureRate"
  Constant38/1 -> Bus Creator1/6  "curveLength"
  Constant39/1 -> Bus Creator1/7  "HeadingAngle"
  Constant43/1 -> Bus Creator1/8  "LateralOffset"
  Constant44/1 -> Bus Creator1/9  "validMaxLongCoordLine"
  Constant1/1 -> Bus Creator1/10  "validMinLongCoordLine"
  Constant2/1 -> Bus Creator1/11  "LineMarkWidth"

== system Grid_SensorLayout_SpatialAllignment_Clustering/SENSOR_MEASUREMENTS/RADAR_CAMERA_EGO_SENSOR_INTERFACE/RoadSensors/LineSensor4/ExtractMeasParam1 ==
  idx : Inport
  time : Inport  Port=2
  Constant : Constant  Value=LINE_CURVATURE_CAM4
  Constant1 : Constant  Value=LINE_CURVDERIVATIVE_CAM4
  Constant2 : Constant  Value=LINE_CURVELENGTH_CAM4
  Constant3 : Constant  Value=LINE_HEADINGANGLE_CAM4
  Constant4 : Constant  Value=LINE_LATERALOFFSET_CAM4
  Constant5 : Constant  Value=LINE_XMIN_CAM4
  Constant6 : Constant  Value=LINE_detTimeStamp_CAM4
  Constant7 : Constant  Value=LINE_XMAX_CAM4
  Constant8 : Constant  Value=LINE_WIDTH_CAM4
  CurvLength : Selector  NumberOfDimensions=2  InputPortWidth=3  IndexOptions=Index vector (port),Index vector (port)  Indices=[1 3],1  OutputSizes=1,1
  Curvature : Selector  NumberOfDimensions=2  InputPortWidth=3  IndexOptions=Index vector (port),Index vector (port)  Indices=[1 3],1  OutputSizes=1,1
  CurvatureRate : Selector  NumberOfDimensions=2  InputPortWidth=3  IndexOptions=Index vector (port),Index vector (port)  Indices=[1 3],1  OutputSizes=1,1
  HeadingAngle : Selector  NumberOfDimensions=2  InputPortWidth=3  IndexOptions=Index vector (port),Index vector (port)  Indices=[1 3],1  OutputSizes=1,1
  LateralOffset : Selector  NumberOfDimensions=2  InputPortWidth=3  IndexOptions=Index vector (port),Index vector (port)  Indices=[1 3],1  OutputSizes=1,1
  lineWidth : Selector  NumberOfDimensions=2  InputPortWidth=3  IndexOptions=Index vector (port),Index vector (port)  Indices=[1 3],1  OutputSizes=1,1
  minValidX : Selector  NumberOfDimensions=2  InputPortWidth=3  IndexOptions=Index vector (port),Index vector (port)  Indices=[1 3],1  OutputSizes=1,1
  minValidY : Selector  NumberOfDimensions=2  InputPortWidth=3  IndexOptions=Index vector (port),Index vector (port)  Indices=[1 3],1  OutputSizes=1,1
  timeStamp : Selector  NumberOfDimensions=2  InputPortWidth=3  IndexOptions=Select all,Index vector (port)  Indices=[1 3],1  OutputSizes=1,1
  curvature : Outport
  curvRate : Outport  Port=2
  curvLength : Outport  Port=3
  headingAngle : Outport  Port=4
  lateralOffset : Outport  Port=5
  xmin : Outport  Port=6
  xmax : Outport  Port=7
  lineMarkWidth : Outport  Port=8
  measCaptureTime : Outport  Port=9
  wires:
  Constant3/1 -> HeadingAngle/1
  Constant2/1 -> CurvLength/1
  HeadingAngle/1 -> headingAngle/1
  Constant/1 -> Curvature/1
  Constant1/1 -> CurvatureRate/1
  CurvLength/1 -> curvLength/1
  Curvature/1 -> curvature/1
  CurvatureRate/1 -> curvRate/1
  Constant4/1 -> LateralOffset/1
  Constant5/1 -> minValidX/1
  Constant6/1 -> timeStamp/1
  timeStamp/1 -> measCaptureTime/1
  minValidX/1 -> xmin/1
  LateralOffset/1 -> lateralOffset/1
  minValidY/1 -> xmax/1
  Constant7/1 -> minValidY/1
  lineWidth/1 -> lineMarkWidth/1
  time/1 -> minValidX/2, minValidY/2, lineWidth/2, timeStamp/2, LateralOffset/2, HeadingAngle/2, CurvLength/2, CurvatureRate/2, Curvature/2
  idx/1 -> minValidX/3, lineWidth/3, minValidY/3, LateralOffset/3, HeadingAngle/3, CurvLength/3, CurvatureRate/3, Curvature/3
  Constant8/1 -> lineWidth/1

== system Grid_SensorLayout_SpatialAllignment_Clustering/SENSOR_MEASUREMENTS/RADAR_CAMERA_EGO_SENSOR_INTERFACE/RoadSensors/LineSensor4/IsValid2 ==
  LineID : Inport
  curvature : Inport  Port=2
  curvatureRate : Inport  Port=3
  curvLength : Inport  Port=4
  HeadingAngle : Inport  Port=5
  Abs{,1..3} (4 alike) : Abs
  Add : Sum  Inputs=++++
  Constant : Constant  Value=uint16(0)
  Data Type Conversion : DataTypeConversion  OutDataTypeStr=uint16
  Switch : Switch  Threshold=0.000001
  validID : Outport
  wires:
  Add/1 -> Switch/2
  Abs2/1 -> Add/3
  Constant/1 -> Switch/3
  Abs/1 -> Add/1
  curvature/1 -> Abs/1
  Abs3/1 -> Add/4
  Abs1/1 -> Add/2
  HeadingAngle/1 -> Abs3/1
  curvatureRate/1 -> Abs1/1
  curvLength/1 -> Abs2/1
  LineID/1 -> Data Type Conversion/1
  Switch/1 -> validID/1
  Data Type Conversion/1 -> Switch/1

== system Grid_SensorLayout_SpatialAllignment_Clustering/SENSOR_MEASUREMENTS/RADAR_CAMERA_EGO_SENSOR_INTERFACE/RoadSensors/LineSensor4/Subsystem1 ==
  CameraLineCoeff : Inport
  curv : Inport  Port=2
  curvRate : Inport  Port=3
  curvLen : Inport  Port=4
  alpha : Inport  Port=5
  ValidID : Inport  Port=6
  lateralOffset : Inport  Port=7
  xmin : Inport  Port=8
  xmax : Inport  Port=9
  lineWidth : Inport  Port=10
  TIME_STAMP : Inport  Port=11
  iter : Inport  Port=12
  Assignment : Assignment  DiagnosticForDimensions=Warning  IndexOptions=Index vector (port)  Indices=1  OutputSizes=1
  Bus Creator1 : BusCreator  Inputs=11  OutDataTypeStr=Bus: LineMeasParam  NonVirtualBus=on
  Bus Creator2 : BusCreator  Inputs=11  OutDataTypeStr=Bus: LineMeasParam  NonVirtualBus=on
  Constant1 : Constant  Value=single(10)
  Constant14 : Constant  Value=uint8(4)
  Constant2 : Constant  Value=single(10)
  Constant{35..39,43} (6 alike) : Constant  Value=single(0)
  Constant44 : Constant  Value=single(10)
  Switch : Switch  Criteria=u2 ~= 0
  C1 : Outport
  wires:
  Bus Creator1/1 -> Switch/3
  ValidID/1 -> Bus Creator1/2, Switch/2, Bus Creator2/2  "lineID"
  Bus Creator2/1 -> Switch/1
  CameraLineCoeff/1 -> Assignment/1
  Switch/1 -> Assignment/2
  iter/1 -> Assignment/3
  Assignment/1 -> C1/1
  TIME_STAMP/1 -> Bus Creator2/1  "TimeStamp"
  curv/1 -> Bus Creator2/4  "curvature"
  curvRate/1 -> Bus Creator2/5  "curvatureRate"
  curvLen/1 -> Bus Creator2/6  "curveLength"
  alpha/1 -> Bus Creator2/7  "HeadingAngle"
  lateralOffset/1 -> Bus Creator2/8  "LateralOffset"
  lineWidth/1 -> Bus Creator2/11  "LineMarkWidth"
  xmax/1 -> Bus Creator2/10  "validMinLongCoordLine"
  xmin/1 -> Bus Creator2/9  "validMaxLongCoordLine"
  Constant35/1 -> Bus Creator1/1  "TimeStamp"
  Constant14/1 -> Bus Creator2/3, Bus Creator1/3  "cameraID"
  Constant36/1 -> Bus Creator1/4  "curvature"
  Constant37/1 -> Bus Creator1/5  "curvatureRate"
  Constant38/1 -> Bus Creator1/6  "curveLength"
  Constant39/1 -> Bus Creator1/7  "HeadingAngle"
  Constant43/1 -> Bus Creator1/8  "LateralOffset"
  Constant44/1 -> Bus Creator1/9  "validMaxLongCoordLine"
  Constant1/1 -> Bus Creator1/10  "validMinLongCoordLine"
  Constant2/1 -> Bus Creator1/11  "LineMarkWidth"

== system Grid_SensorLayout_SpatialAllignment_Clustering/SENSOR_MEASUREMENTS/RADAR_CAMERA_EGO_SENSOR_INTERFACE/RoadSensors/LineSensor5/ExtractMeasParam1 ==
  idx : Inport
  time : Inport  Port=2
  Constant : Constant  Value=LINE_CURVATURE_CAM5
  Constant1 : Constant  Value=LINE_CURVDERIVATIVE_CAM5
  Constant2 : Constant  Value=LINE_CURVELENGTH_CAM5
  Constant3 : Constant  Value=LINE_HEADINGANGLE_CAM5
  Constant4 : Constant  Value=LINE_LATERALOFFSET_CAM5
  Constant5 : Constant  Value=LINE_XMIN_CAM5
  Constant6 : Constant  Value=LINE_detTimeStamp_CAM5
  Constant7 : Constant  Value=LINE_XMAX_CAM5
  Constant8 : Constant  Value=LINE_WIDTH_CAM5
  CurvLength : Selector  NumberOfDimensions=2  InputPortWidth=3  IndexOptions=Index vector (port),Index vector (port)  Indices=[1 3],1  OutputSizes=1,1
  Curvature : Selector  NumberOfDimensions=2  InputPortWidth=3  IndexOptions=Index vector (port),Index vector (port)  Indices=[1 3],1  OutputSizes=1,1
  CurvatureRate : Selector  NumberOfDimensions=2  InputPortWidth=3  IndexOptions=Index vector (port),Index vector (port)  Indices=[1 3],1  OutputSizes=1,1
  HeadingAngle : Selector  NumberOfDimensions=2  InputPortWidth=3  IndexOptions=Index vector (port),Index vector (port)  Indices=[1 3],1  OutputSizes=1,1
  LateralOffset : Selector  NumberOfDimensions=2  InputPortWidth=3  IndexOptions=Index vector (port),Index vector (port)  Indices=[1 3],1  OutputSizes=1,1
  lineWidth : Selector  NumberOfDimensions=2  InputPortWidth=3  IndexOptions=Index vector (port),Index vector (port)  Indices=[1 3],1  OutputSizes=1,1
  minValidX : Selector  NumberOfDimensions=2  InputPortWidth=3  IndexOptions=Index vector (port),Index vector (port)  Indices=[1 3],1  OutputSizes=1,1
  minValidY : Selector  NumberOfDimensions=2  InputPortWidth=3  IndexOptions=Index vector (port),Index vector (port)  Indices=[1 3],1  OutputSizes=1,1
  timeStamp : Selector  NumberOfDimensions=2  InputPortWidth=3  IndexOptions=Select all,Index vector (port)  Indices=[1 3],1  OutputSizes=1,1
  curvature : Outport
  curvRate : Outport  Port=2
  curvLength : Outport  Port=3
  headingAngle : Outport  Port=4
  lateralOffset : Outport  Port=5
  xmin : Outport  Port=6
  xmax : Outport  Port=7
  lineMarkWidth : Outport  Port=8
  measCaptureTime : Outport  Port=9
  wires:
  Constant3/1 -> HeadingAngle/1
  Constant2/1 -> CurvLength/1
  HeadingAngle/1 -> headingAngle/1
  Constant/1 -> Curvature/1
  Constant1/1 -> CurvatureRate/1
  CurvLength/1 -> curvLength/1
  Curvature/1 -> curvature/1
  CurvatureRate/1 -> curvRate/1
  Constant4/1 -> LateralOffset/1
  Constant5/1 -> minValidX/1
  Constant6/1 -> timeStamp/1
  timeStamp/1 -> measCaptureTime/1
  minValidX/1 -> xmin/1
  LateralOffset/1 -> lateralOffset/1
  minValidY/1 -> xmax/1
  Constant7/1 -> minValidY/1
  lineWidth/1 -> lineMarkWidth/1
  time/1 -> minValidX/2, minValidY/2, lineWidth/2, timeStamp/2, LateralOffset/2, HeadingAngle/2, CurvLength/2, CurvatureRate/2, Curvature/2
  idx/1 -> minValidX/3, lineWidth/3, minValidY/3, LateralOffset/3, HeadingAngle/3, CurvLength/3, CurvatureRate/3, Curvature/3
  Constant8/1 -> lineWidth/1

== system Grid_SensorLayout_SpatialAllignment_Clustering/SENSOR_MEASUREMENTS/RADAR_CAMERA_EGO_SENSOR_INTERFACE/RoadSensors/LineSensor5/IsValid2 ==
  LineID : Inport
  curvature : Inport  Port=2
  curvatureRate : Inport  Port=3
  curvLength : Inport  Port=4
  HeadingAngle : Inport  Port=5
  Abs{,1..3} (4 alike) : Abs
  Add : Sum  Inputs=++++
  Constant : Constant  Value=uint16(0)
  Data Type Conversion : DataTypeConversion  OutDataTypeStr=uint16
  Switch : Switch  Threshold=0.000001
  validID : Outport
  wires:
  Add/1 -> Switch/2
  Abs2/1 -> Add/3
  Constant/1 -> Switch/3
  Abs/1 -> Add/1
  curvature/1 -> Abs/1
  Abs3/1 -> Add/4
  Abs1/1 -> Add/2
  HeadingAngle/1 -> Abs3/1
  curvatureRate/1 -> Abs1/1
  curvLength/1 -> Abs2/1
  LineID/1 -> Data Type Conversion/1
  Switch/1 -> validID/1
  Data Type Conversion/1 -> Switch/1

== system Grid_SensorLayout_SpatialAllignment_Clustering/SENSOR_MEASUREMENTS/RADAR_CAMERA_EGO_SENSOR_INTERFACE/RoadSensors/LineSensor5/Subsystem1 ==
  CameraLineCoeff : Inport
  curv : Inport  Port=2
  curvRate : Inport  Port=3
  curvLen : Inport  Port=4
  alpha : Inport  Port=5
  ValidID : Inport  Port=6
  lateralOffset : Inport  Port=7
  xmin : Inport  Port=8
  xmax : Inport  Port=9
  lineWidth : Inport  Port=10
  TIME_STAMP : Inport  Port=11
  iter : Inport  Port=12
  Assignment : Assignment  DiagnosticForDimensions=Warning  IndexOptions=Index vector (port)  Indices=1  OutputSizes=1
  Bus Creator1 : BusCreator  Inputs=11  OutDataTypeStr=Bus: LineMeasParam  NonVirtualBus=on
  Bus Creator2 : BusCreator  Inputs=11  OutDataTypeStr=Bus: LineMeasParam  NonVirtualBus=on
  Constant1 : Constant  Value=single(10)
  Constant14 : Constant  Value=uint8(5)
  Constant2 : Constant  Value=single(10)
  Constant{35..39,43} (6 alike) : Constant  Value=single(0)
  Constant44 : Constant  Value=single(10)
  Switch : Switch  Criteria=u2 ~= 0
  C1 : Outport
  wires:
  Bus Creator1/1 -> Switch/3
  ValidID/1 -> Bus Creator1/2, Switch/2, Bus Creator2/2  "lineID"
  Bus Creator2/1 -> Switch/1
  CameraLineCoeff/1 -> Assignment/1
  Switch/1 -> Assignment/2
  iter/1 -> Assignment/3
  Assignment/1 -> C1/1
  TIME_STAMP/1 -> Bus Creator2/1  "TimeStamp"
  curv/1 -> Bus Creator2/4  "curvature"
  curvRate/1 -> Bus Creator2/5  "curvatureRate"
  curvLen/1 -> Bus Creator2/6  "curveLength"
  alpha/1 -> Bus Creator2/7  "HeadingAngle"
  lateralOffset/1 -> Bus Creator2/8  "LateralOffset"
  lineWidth/1 -> Bus Creator2/11  "LineMarkWidth"
  xmax/1 -> Bus Creator2/10  "validMinLongCoordLine"
  xmin/1 -> Bus Creator2/9  "validMaxLongCoordLine"
  Constant35/1 -> Bus Creator1/1  "TimeStamp"
  Constant14/1 -> Bus Creator2/3, Bus Creator1/3  "cameraID"
  Constant36/1 -> Bus Creator1/4  "curvature"
  Constant37/1 -> Bus Creator1/5  "curvatureRate"
  Constant38/1 -> Bus Creator1/6  "curveLength"
  Constant39/1 -> Bus Creator1/7  "HeadingAngle"
  Constant43/1 -> Bus Creator1/8  "LateralOffset"
  Constant44/1 -> Bus Creator1/9  "validMaxLongCoordLine"
  Constant1/1 -> Bus Creator1/10  "validMinLongCoordLine"
  Constant2/1 -> Bus Creator1/11  "LineMarkWidth"

== system Grid_SensorLayout_SpatialAllignment_Clustering/SENSOR_MEASUREMENTS/RADAR_CAMERA_EGO_SENSOR_INTERFACE/RoadSensors/LineSensor6/ExtractMeasParam1 ==
  idx : Inport
  time : Inport  Port=2
  Constant : Constant  Value=LINE_CURVATURE_CAM6
  Constant1 : Constant  Value=LINE_CURVDERIVATIVE_CAM6
  Constant2 : Constant  Value=LINE_CURVELENGTH_CAM6
  Constant3 : Constant  Value=LINE_HEADINGANGLE_CAM6
  Constant4 : Constant  Value=LINE_LATERALOFFSET_CAM6
  Constant5 : Constant  Value=LINE_XMIN_CAM6
  Constant6 : Constant  Value=LINE_detTimeStamp_CAM6
  Constant7 : Constant  Value=LINE_XMAX_CAM6
  Constant8 : Constant  Value=LINE_WIDTH_CAM6
  CurvLength : Selector  NumberOfDimensions=2  InputPortWidth=3  IndexOptions=Index vector (port),Index vector (port)  Indices=[1 3],1  OutputSizes=1,1
  Curvature : Selector  NumberOfDimensions=2  InputPortWidth=3  IndexOptions=Index vector (port),Index vector (port)  Indices=[1 3],1  OutputSizes=1,1
  CurvatureRate : Selector  NumberOfDimensions=2  InputPortWidth=3  IndexOptions=Index vector (port),Index vector (port)  Indices=[1 3],1  OutputSizes=1,1
  HeadingAngle : Selector  NumberOfDimensions=2  InputPortWidth=3  IndexOptions=Index vector (port),Index vector (port)  Indices=[1 3],1  OutputSizes=1,1
  LateralOffset : Selector  NumberOfDimensions=2  InputPortWidth=3  IndexOptions=Index vector (port),Index vector (port)  Indices=[1 3],1  OutputSizes=1,1
  lineWidth : Selector  NumberOfDimensions=2  InputPortWidth=3  IndexOptions=Index vector (port),Index vector (port)  Indices=[1 3],1  OutputSizes=1,1
  minValidX : Selector  NumberOfDimensions=2  InputPortWidth=3  IndexOptions=Index vector (port),Index vector (port)  Indices=[1 3],1  OutputSizes=1,1
  minValidY : Selector  NumberOfDimensions=2  InputPortWidth=3  IndexOptions=Index vector (port),Index vector (port)  Indices=[1 3],1  OutputSizes=1,1
  timeStamp : Selector  NumberOfDimensions=2  InputPortWidth=3  IndexOptions=Select all,Index vector (port)  Indices=[1 3],1  OutputSizes=1,1
  curvature : Outport
  curvRate : Outport  Port=2
  curvLength : Outport  Port=3
  headingAngle : Outport  Port=4
  lateralOffset : Outport  Port=5
  xmin : Outport  Port=6
  xmax : Outport  Port=7
  lineMarkWidth : Outport  Port=8
  measCaptureTime : Outport  Port=9
  wires:
  Constant3/1 -> HeadingAngle/1
  Constant2/1 -> CurvLength/1
  HeadingAngle/1 -> headingAngle/1
  Constant/1 -> Curvature/1
  Constant1/1 -> CurvatureRate/1
  CurvLength/1 -> curvLength/1
  Curvature/1 -> curvature/1
  CurvatureRate/1 -> curvRate/1
  Constant4/1 -> LateralOffset/1
  Constant5/1 -> minValidX/1
  Constant6/1 -> timeStamp/1
  timeStamp/1 -> measCaptureTime/1
  minValidX/1 -> xmin/1
  LateralOffset/1 -> lateralOffset/1
  minValidY/1 -> xmax/1
  Constant7/1 -> minValidY/1
  lineWidth/1 -> lineMarkWidth/1
  time/1 -> minValidX/2, minValidY/2, lineWidth/2, timeStamp/2, LateralOffset/2, HeadingAngle/2, CurvLength/2, CurvatureRate/2, Curvature/2
  idx/1 -> minValidX/3, lineWidth/3, minValidY/3, LateralOffset/3, HeadingAngle/3, CurvLength/3, CurvatureRate/3, Curvature/3
  Constant8/1 -> lineWidth/1

== system Grid_SensorLayout_SpatialAllignment_Clustering/SENSOR_MEASUREMENTS/RADAR_CAMERA_EGO_SENSOR_INTERFACE/RoadSensors/LineSensor6/IsValid2 ==
  LineID : Inport
  curvature : Inport  Port=2
  curvatureRate : Inport  Port=3
  curvLength : Inport  Port=4
  HeadingAngle : Inport  Port=5
  Abs{,1..3} (4 alike) : Abs
  Add : Sum  Inputs=++++
  Constant : Constant  Value=uint16(0)
  Data Type Conversion : DataTypeConversion  OutDataTypeStr=uint16
  Switch : Switch  Threshold=0.000001
  validID : Outport
  wires:
  Add/1 -> Switch/2
  Abs2/1 -> Add/3
  Constant/1 -> Switch/3
  Abs/1 -> Add/1
  curvature/1 -> Abs/1
  Abs3/1 -> Add/4
  Abs1/1 -> Add/2
  HeadingAngle/1 -> Abs3/1
  curvatureRate/1 -> Abs1/1
  curvLength/1 -> Abs2/1
  LineID/1 -> Data Type Conversion/1
  Switch/1 -> validID/1
  Data Type Conversion/1 -> Switch/1
